simulink model "HardwareInteg_v3"  (R2023a)
settings: Solver=VariableStepAuto  StartTime=0.0  StopTime=inf  FixedStep=0.01  RelTol=1e-3
model workspace (MAT data in the model file):
  D = 0
  I = 0
  N = 100
  P = 1
  setpoint = 1
undefined symbols (not defined in the file or in its folder): daq
libraries: sldrtlib x2, dspstat3 x2, daqlib x2, visionsinks x1
settings Model: Creator=Siril TD  LastModifiedBy=Siril TD
settings OptimizationCC: DefaultParameterBehavior=Inlined  EnhancedBackFolding=on  PassReuseOutputArgsThreshold=0  OptimizeBlockOrder=speed  DifferentSizesBufferReuse=on
settings DebuggingCC: ParameterTunabilityLossMsg=error
settings HardwareCC: TargetBitPerPointer=64  TargetBitPerSizeT=64  TargetBitPerPtrDiffT=64  TargetLongLongMode=on  TargetIntDivRoundTo=Zero  TargetEndianess=LittleEndian  TargetWordSize=64  TargetHWDeviceType=MATLAB Host  ProdEqTarget=off
settings SFSimCC: SimGenImportedTypeDefs=on  SimTargetLang=C++
settings RTWCC: GenCodeOnly=on
settings CodeAppCC: ForceParamTrailComments=on  MaxIdLength=63  OperatorAnnotations=on

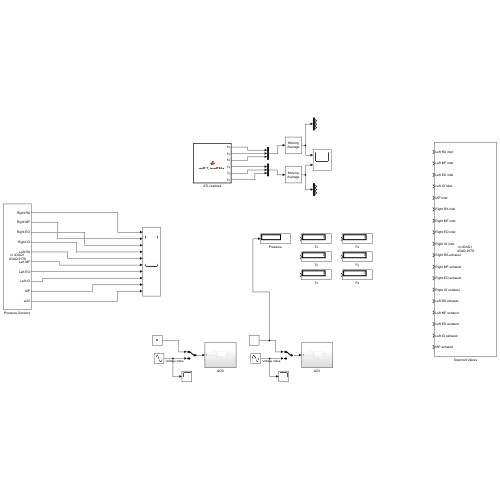
[thumbnail: Simulink's stored preview of the top-level diagram]
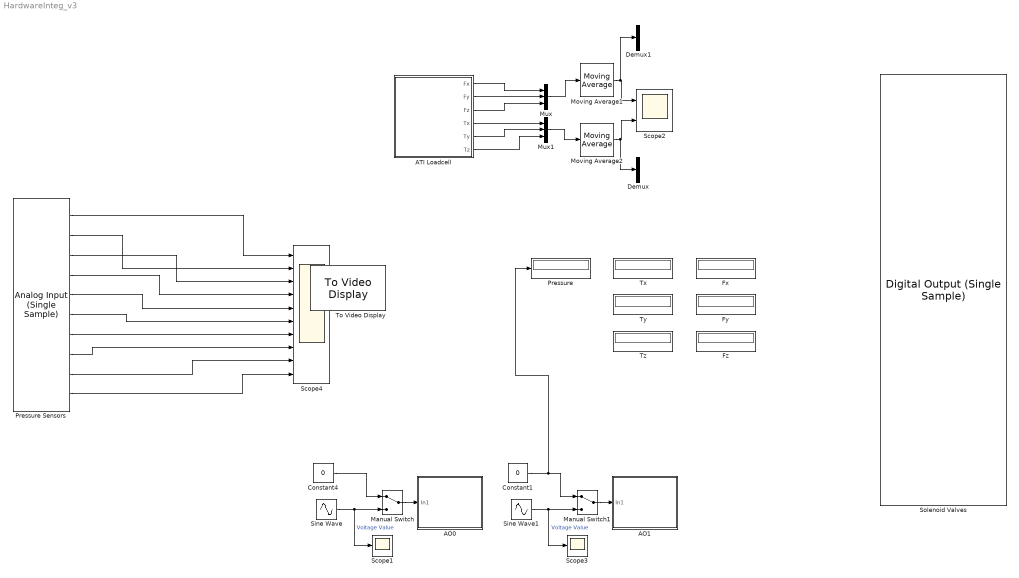
== system HardwareInteg_v3 ==
  AO0 : Subsystem
  AO1 : Subsystem
  ATI Loadcell : MATLAB Function  TreatAsAtomicUnit=on
  Constant1 : Constant  Value=0
  Constant4 : Constant  Value=0
  Demux : Demux  Outputs=3
  Demux1 : Demux  Outputs=3
  Fx : Display
  Fy : Display
  Fz : Display
  Manual Switch : ManualSwitch
  Manual Switch1 : ManualSwitch
  Moving Average1 : dspstat3/Moving Average  Method=Sliding window  ForgettingFactorPort=off  SpecifyWindowLength=on  WindowLength=4  OverlapLength=3  AllowArbitraryInputLength=off  ForgettingFactor=0.9  SimulateUsing=Code generation
  Moving Average2 : dspstat3/Moving Average  Method=Sliding window  ForgettingFactorPort=off  SpecifyWindowLength=on  WindowLength=4  OverlapLength=3  AllowArbitraryInputLength=off  ForgettingFactor=0.9  SimulateUsing=Code generation
  Mux : Mux  Inputs=3
  Mux1 : Mux  Inputs=3
  Pressure : Display
  Pressure Sensors : daqlib/Analog Input (Single Sample)  DeviceMenu=ni cDAQ1 (cDAQ-9178)  Device=ni cDAQ1 (cDAQ-9178)  ModuleInfo=cDAQ1Mod1(NI 9205)  ObjConstructor=daq.createSession('ni')  BlockSampleTime=0.001  NChannelsSelected=10  Channels=0$ai0$$cDAQ1Mod1$1$4$1$1$#1$ai1$Right RA$cDAQ1Mod1$1$4$1$1$#1$ai2$Right MF$cDAQ1Mod1$1$4$1$1$#1$ai3$Right EO$cDAQ1Mod1$1$4$1$1$#1$ai4$Right IO$cDAQ1Mod1$1$4$1$1$#1$ai5$Left RA$cDAQ1Mod1$1$4$1$1$#1$ai6$Left MF$cDAQ1Mod1$1$4$1$1$#1$ai7$Left EO$cDAQ1Mod1$1$4$1$1$#1$ai8$Left IO$cDAQ1Mod1$1$4$1$1$#1$ai9$IAP$cDAQ1Mod1$1$4$1$1$#1$ai10$$cDAQ1Mod1$1$4$1$1$#0$ai11$$cDAQ1Mod1$1$4$1$1$#0$ai12$$cDAQ1Mod1$1$4$1$1$#0$ai13$$cDAQ1Mod1$1$4$1$1$#0$ai14$$cDAQ1Mod1$1$4$1$1$#0$ai15$$cDAQ1Mod1$1$4$1$1$#0$ai16$$cDAQ1Mod1$1$4$3$1$#0$ai17$$cDAQ1Mod1$1$4$3$1$#0$ai18$$cDAQ1Mod1$1$4$3$1$#0$ai19$$cDAQ1Mod1$1$4$3$1$#0$ai20$$cDAQ1Mod1$1$4$3$1$#0$ai21$$cDAQ1Mod1$1$4$3$1$#0$ai22$$cDAQ1Mod1$1$4$3$1$#0$ai23$$cDAQ1Mod1$1$4$3$1$#0$ai24$$cDAQ1Mod1$1$4$1$1$#0$ai25$$cDAQ1Mod1$1$4$1$1$#0$ai26$$cDAQ1Mod1$1$4$1$1$#0$ai27$$cDAQ1Mod1$1$4$1$1$#0$ai28$$cDAQ1Mod1$1$4$1$1$#0$ai29$$cDAQ1Mod1$1$4$1$1$#0$ai30$$cDAQ1Mod1$1$4$1$1$#0$ai31$$cDAQ1Mod1$1$4$1$1$#  NPorts=1 per channel  OutputTimestamp=off
  Scope1 : Scope
  Scope2 : Scope  NumInputPorts=2
  Scope3 : Scope
  Scope4 : Scope  NumInputPorts=10
  Sine Wave : Sin  Amplitude=2.5  Bias=2.5  Frequency=0.1  SampleTime=0
  Sine Wave1 : Sin  Amplitude=2.5  Bias=2.5  Frequency=0.5  SampleTime=0
  Solenoid Valves : daqlib/Digital Output (Single Sample)  DeviceMenu=ni cDAQ1 (cDAQ-9178)  Device=ni cDAQ1 (cDAQ-9178)  ModuleInfo=cDAQ1Mod3(NI 9485)cDAQ1Mod4(NI 9485)cDAQ1Mod5(NI 9485)cDAQ1Mod6(NI 9485)  ObjConstructor=daq.createSession('ni')  BlockSampleTime=0.001  IsDigitalInput=off  NLinesSelected=18  Lines=0$port0/line0$$cDAQ1Mod3$#1$port0/line1$Left RA inlet$cDAQ1Mod3$#1$port0/line2$Left MF inlet$cDAQ1Mod3$#1$port0/line3$Left EO inlet$cDAQ1Mod3$#1$port0/line4$Left IO inlet$cDAQ1Mod3$#1$port0/line5$IAP inlet$cDAQ1Mod3$#0$port0/line6$$cDAQ1Mod3$#0$port0/line7$$cDAQ1Mod3$#0$port0/line0$$cDAQ1Mod4$#1$port0/line1$Right RA inlet$cDAQ1Mod4$#0$port0/line2$$cDAQ1Mod4$#1$port0/line3$Right MF inlet$cDAQ1Mod4$#0$port0/line4$$cDAQ1Mod4$#1$port0/line5$Right EO inlet$cDAQ1Mod4$#1$port0/line6$Right IO inlet$cDAQ1Mod4$#0$port0/line7$$cDAQ1Mod4$#0$port0/line0$$cDAQ1Mod5$#1$port0/line1$Right RA exhaust$cDAQ1Mod5$#0$port0/line2$$cDAQ1Mod5$#1$port0/line3$Right MF exhaust$cDAQ1Mod5$#0$port0/line4$$cDAQ1Mod5$#1$port0/line5$Right EO exhaust$cDAQ1Mod5$#1$port0/line6$Right IO exhaust$cDAQ1Mod5$#0$port0/line7$$cDAQ1Mod5$#0$port0/line0$$cDAQ1Mod6$#1$port0/line1$Left RA exhaust$cDAQ1Mod6$#1$port0/line2$Left MF exhaust$cDAQ1Mod6$#1$port0/line3$Left EO exhaust$cDAQ1Mod6$#1$port0/line4$Left IO exhaust$cDAQ1Mod6$#1$port0/line5$IAP exhaust$cDAQ1Mod6$#0$port0/line6$$cDAQ1Mod6$#0$port0/line7$$cDAQ1Mod6$#  NPorts=1 per line
  Tx : Display
  Ty : Display
  Tz : Display
  To Video Display : visionsinks/To Video Display  IOType=viewer  windowSizeMode=True size (1:1)  openAtMdlStart=on  fullScreen=off  videoWindowX=44  videoWindowY=41  saveWindowSize=off  videoWindowWidth=44  videoWindowHeight=41  inputColorFormat=RGB  inputType=Obsolete  imagePorts=One multidimensional signal  OutputDevice=On-screen video monitor  dataOrg=Column-major  isWindowOpen=off
      settings: LibrarySourceBlock=vipviewers_win32/To Video Display
  wires:
  Pressure Sensors/1 -> Scope4/1
  ATI Loadcell/1(Fx) -> Mux/1
  ATI Loadcell/2(Fy) -> Mux/2
  ATI Loadcell/3(Fz) -> Mux/3
  ATI Loadcell/4(Tx) -> Mux1/1
  ATI Loadcell/5(Ty) -> Mux1/2
  ATI Loadcell/6(Tz) -> Mux1/3
  Mux/1 -> Moving Average1/1
  Moving Average1/1 -> Demux1/1, Scope2/1
  Mux1/1 -> Moving Average2/1
  Moving Average2/1 -> Demux/1, Scope2/2
  Pressure Sensors/3 -> Scope4/3
  Pressure Sensors/4 -> Scope4/4
  Pressure Sensors/5 -> Scope4/5
  Pressure Sensors/6 -> Scope4/6
  Pressure Sensors/7 -> Scope4/7
  Pressure Sensors/8 -> Scope4/8
  Pressure Sensors/9 -> Scope4/9
  Pressure Sensors/10 -> Scope4/10
  Pressure Sensors/2 -> Scope4/2
  Constant4/1 -> Manual Switch/1
  Sine Wave/1 -> Scope1/1, Manual Switch/2  "Voltage Value"
  Manual Switch/1 -> AO0/1(In1)
  Sine Wave1/1 -> Scope3/1, Manual Switch1/2  "Voltage Value"
  Constant1/1 -> Manual Switch1/1, Pressure/1
  Manual Switch1/1 -> AO1/1(In1)

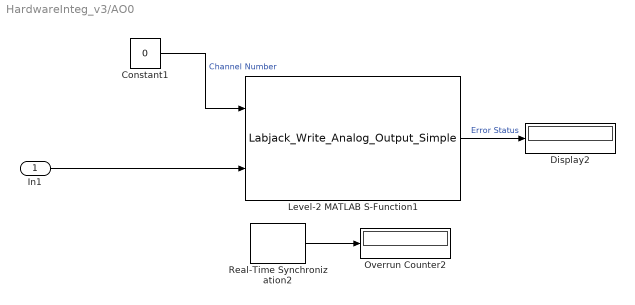
== system HardwareInteg_v3/AO0 ==
  In1 : Inport
  Constant1 : Constant  Value=0
  Display2 : Display
  Level-2 MATLAB S-Function1 : M-S-Function  FunctionName=Labjack_Write_Analog_Output_Simple
  Overrun Counter2 : Display
  Real-Time Synchronization2 : sldrtlib/Real-Time Synchronization  SampleTime=0.1  MaxMissedTicks=100  ShowMissedTicks=on  YieldWhenWaiting=off
  wires:
  In1/1 -> Level-2 MATLAB S-Function1/2
  Constant1/1 -> Level-2 MATLAB S-Function1/1  "Channel Number"
  Real-Time Synchronization2/1 -> Overrun Counter2/1
  Level-2 MATLAB S-Function1/1 -> Display2/1  "Error Status"

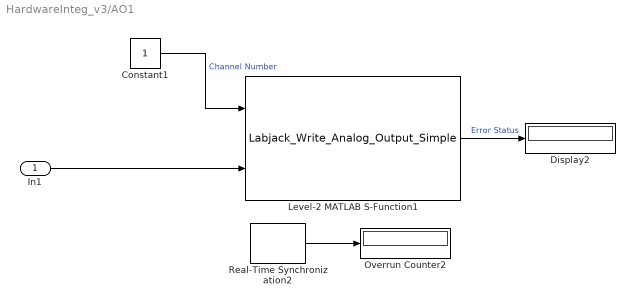
== system HardwareInteg_v3/AO1 ==
  In1 : Inport
  Constant1 : Constant
  Display2 : Display
  Level-2 MATLAB S-Function1 : M-S-Function  FunctionName=Labjack_Write_Analog_Output_Simple
  Overrun Counter2 : Display
  Real-Time Synchronization2 : sldrtlib/Real-Time Synchronization  SampleTime=0.1  MaxMissedTicks=100  ShowMissedTicks=on  YieldWhenWaiting=off
  wires:
  In1/1 -> Level-2 MATLAB S-Function1/2
  Constant1/1 -> Level-2 MATLAB S-Function1/1  "Channel Number"
  Real-Time Synchronization2/1 -> Overrun Counter2/1
  Level-2 MATLAB S-Function1/1 -> Display2/1  "Error Status"

== matlab function HardwareInteg_v3/ATI Loadcell ==
  data: Fx output; Fy output; Fz output; Tx output; Ty output; Tz output
function [Fx, Fy, Fz, Tx, Ty, Tz] = netFT_readData()
    % Declare the extrinsic wrapper function
    coder.extrinsic('ATI_Wrapper');  % Tell Simulink that myWrapper is an external function

    % Initialize output variables as numeric types
    Fx = 0;
    Fy = 0;
    Fz = 0;
    Tx = 0;
    Ty = 0;
    Tz = 0;

    % Call the wrapper function
    [Fx, Fy, Fz, Tx, Ty, Tz] = ATI_Wrapper();  % Get the force and torque data
end
